simulink library "Pitch_Functions"  (Simulink 6.5)
undefined symbols (not defined in the file or in its folder): A, ABS, B, C, D, P_PitchProfilerAccLim, P_PitchProfilerMaxGain, P_PitchProfilerPostDelay, P_PitchProfilerPreDelay, P_PitchProfilerSpdLim, P_PitchProfilerTc, P_PitchProfilerTcRatio, P_PitchSpinningPos, PITCH_CYCLE_TIME, RND, SQR
libraries: StandardLib x187, WindLib x15, Pitch_Functions x6, simulink x4
(part 2 of 3)

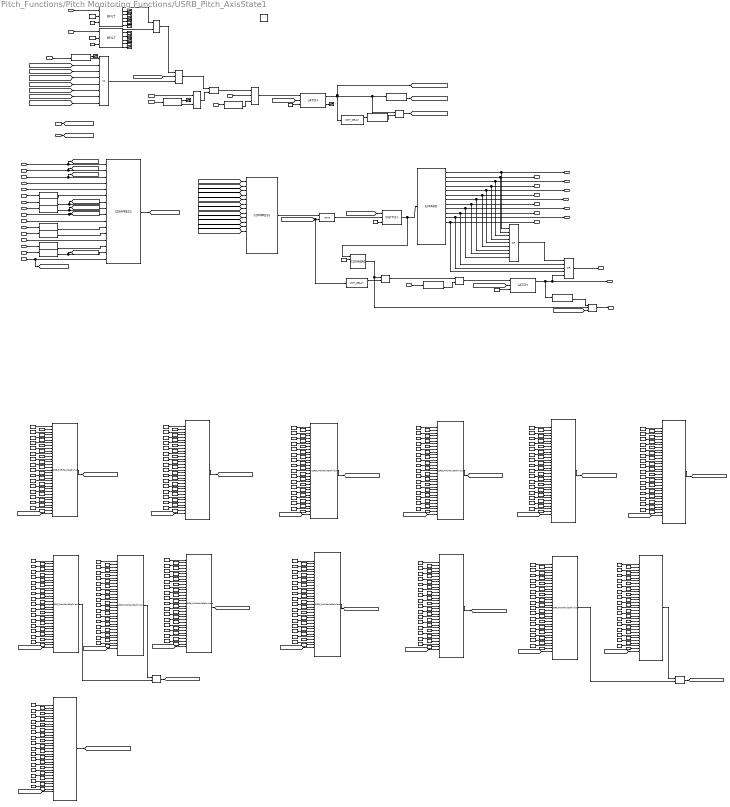
== system Pitch_Functions/Pitch Monitoring Functions/USRB_Pitch_AxisState1 ==
  note: Fault 11
  note: Fault 10
  note: Fault 9
  note: Fault 8
  note: Fault 7
  note: Fault 6
  note: Fault 5
  note: Fault 4
  note: Fault 3
  note: Fault 2
  note: Fault 1
  note: Fault 12
  B_In_SafetyLoopClosed : Inport  DataType=boolean
  DO_OpCtl_TbPitchRectifierOn : Inport  Port=2  DataType=boolean
  B_Pitch_ConverterReady : Inport  Port=3  DataType=boolean
  B_ResetLatch : Inport  Port=4  DataType=boolean
  B_EnableThyristorFault : Inport  Port=5  DataType=boolean
  B_Pitch_PitchThysitor : Inport  Port=6  DataType=boolean
  DI_In_PitchCtrlReady : Inport  Port=7  DataType=boolean
  DI_In_SpeedLoss : Inport  Port=8  DataType=boolean
  DI_In_MarkerLoss : Inport  Port=9  DataType=boolean
  DI_In_IncEncCorrection : Inport  Port=10  DataType=boolean
  DI_In_LS90AngleErr : Inport  Port=11  DataType=boolean
  DI_In_BatDCMCtr : Inport  Port=12  DataType=boolean
  DI_In_DCLinkOK : Inport  Port=13  DataType=boolean
  DI_In_BrakeOK : Inport  Port=14  DataType=boolean
  DI_In_FieldOK : Inport  Port=15  DataType=boolean
  DI_In_OverSpeed : Inport  Port=16  DataType=boolean
  DI_In_SpeedProfileFault : Inport  Port=17  DataType=boolean
  DI_In_SafetyRelayPLC : Inport  Port=18  DataType=boolean
  DI_In_CvrtDCMCtr : Inport  Port=19  DataType=boolean
  DI_In_LVRTAmpHourTrip : Inport  Port=20  DataType=boolean
  DI_In_PICCommOK : Inport  Port=21  DataType=boolean
  DI_In_PhaseOk : Inport  Port=22  DataType=boolean
  DI_In_CommunAEPAx_Ok : Inport  Port=23  DataType=boolean
  SM_Pitch_IOLinkAxisXFault : Inport  Port=24  DataType=boolean
  DI_In_ConverterFaulted : Inport  Port=25  DataType=boolean
  SM_Pitch_AxisxCtlUnitERR : Inport  Port=26  DataType=boolean
  1700ms : Constant  Value=1700  OutDataTypeMode=uint32  OutDataType=sfix(16)  ConRadixGroup=Use specified scaling  OutScaling=2^0  SampleTime=inf  FramePeriod=inf
  2h{1,19,30,32,34,36,40..43,45..46,48..58,60..61,63..71,74,76..78,81,83,88,91,94..95,97..98,100..106,108..109,112..118,120,126,132,134,137,140..141,143..144,146..152,154,168..169,171,174..175,177..178,180..183,185,195,198..199,202,205..209,214..222,224,226,229..235,237..238,240,248,253,256,259..264,266..273,275,280,282,290,292,294,297..301,305,307..312,326,337,342..346,348,364..365,368,372..376,384,386..387,390..393,398,405,409..410,412..416,418..424,426,431,438,440,443,446..450,486..492,494,505,508,511,514..515,517..518} (220 alike) : Constant  Value=1  OutDataTypeMode=boolean  OutDataType=sfix(16)  ConRadixGroup=Use specified scaling  OutScaling=2^0  SampleTime=inf  FramePeriod=inf
  2h{2..5,7..10,12..18,20..22,24..29,31,33,35,37..39,44,47,59,62,72..73,75,79,82,84..87,89..90,92..93,96,99,107,110..111,119,121..125,127..131,133,135..136,138..139,142,145,153,155..167,170,172..173,176,179,184,186..194,196..197,200..201,203..204,210..213,223,225,227..228,236,239,241..247,249..252,254..255,257..258,265,274,276..279,281,283..289,291,293,295..296,302..304,306,313..314,325,347,349,351..355,357..358,360..363,366..367,369..371,377..383,385,388..389,394..395,397,399..404,406..408,411,417,425,428..430,433..437,439,441..442,444..445,451..452,493,496..499,501..504,506..507,509..510,512..513,516,519} (230 alike) : Constant  Value=0  OutDataTypeMode=boolean  OutDataType=sfix(16)  ConRadixGroup=Use specified scaling  OutScaling=2^0  SampleTime=inf  FramePeriod=inf
  2h11 : Constant  Value=0  OutDataTypeMode=uint32  OutDataType=sfix(16)  ConRadixGroup=Use specified scaling  OutScaling=2^0  SampleTime=inf  FramePeriod=inf
  2h23 : Constant  Value=0  OutDataTypeMode=uint16  OutDataType=sfix(16)  ConRadixGroup=Use specified scaling  OutScaling=2^0  SampleTime=inf  FramePeriod=inf
  2h6 : Constant  Value=0  OutDataTypeMode=uint16  OutDataType=sfix(16)  ConRadixGroup=Use specified scaling  OutScaling=2^0  SampleTime=inf  FramePeriod=inf
  2h80 : Constant  Value=0  OutDataTypeMode=uint32  OutDataType=sfix(16)  ConRadixGroup=Use specified scaling  OutScaling=2^0  SampleTime=inf  FramePeriod=inf
  700ms : Constant  Value=700  OutDataTypeMode=uint32  OutDataType=sfix(16)  ConRadixGroup=Use specified scaling  OutScaling=2^0  SampleTime=inf  FramePeriod=inf
  AND{1..2,5,7,9} (5 alike) : StandardLib/Logical operations/AND  RepeatCnt=1  SampleTime=-1  ExecutionOrder=0
  AND10 : StandardLib/Logical operations/AND  RepeatCnt=2  SampleTime=-1  ExecutionOrder=0
  AND6 : StandardLib/Logical operations/AND  RepeatCnt=2  SampleTime=-1  ExecutionOrder=0
  AND8 : StandardLib/Logical operations/AND  RepeatCnt=2  SampleTime=-1  ExecutionOrder=0
  BFILT1 : StandardLib/Filters/BFILT  SampleTime=-1  ExecutionOrder=0
  BFILT3 : StandardLib/Filters/BFILT  SampleTime=-1  ExecutionOrder=0
  COMPARE : StandardLib/Math operations/COMPARE  Equation===  DataType=UINT16  SampleTime=-1  ExecutionOrder=0
  COMPRESS : StandardLib/Memory operations/COMPRESS  RepeatCnt=16  SampleTime=-1  ExecutionOrder=0
  COMPRESS4 : StandardLib/Memory operations/COMPRESS  RepeatCnt=16  SampleTime=-1  ExecutionOrder=0
  DocBlock1 : simulink/Model-Wide Utilities/DocBlock  SystemSampleTime=-1  DocumentType=Text
  EXPAND : StandardLib/Memory operations/EXPAND  SampleTime=-1  ExecutionOrder=0
  LATCH2 : StandardLib/Logical operations/LATCH  SampleTime=-1  ExecutionOrder=0
  LATCH3 : StandardLib/Logical operations/LATCH  SampleTime=-1  ExecutionOrder=0
  MOVE : StandardLib/Memory operations/MOVE  DataType=UINT16  SampleTime=-1  ExecutionOrder=0
  NOT{,1,3..11,13..15} (14 alike) : StandardLib/Logical operations/NOT  SampleTime=-1  ExecutionOrder=0
  OR : StandardLib/Logical operations/OR  RepeatCnt=1  SampleTime=-1  ExecutionOrder=0
  OR1 : StandardLib/Logical operations/OR  RepeatCnt=1  SampleTime=-1  ExecutionOrder=0
  OR2 : StandardLib/Logical operations/OR  RepeatCnt=1  SampleTime=-1  ExecutionOrder=0
  OR3 : StandardLib/Logical operations/OR  RepeatCnt=7  SampleTime=-1  ExecutionOrder=0
  OR4 : StandardLib/Logical operations/OR  RepeatCnt=8  SampleTime=-1  ExecutionOrder=0
  OR5 : StandardLib/Logical operations/OR  RepeatCnt=4  SampleTime=-1  ExecutionOrder=0
  SWITCH1 : StandardLib/Memory operations/SWITCH  DataType=UINT16  SampleTime=-1  ExecutionOrder=0
  Terminator{1..13} (13 alike) : Terminator
  UNIT_DELAY : StandardLib/Memory operations/UNIT_DELAY  DataType=BOOLEAN  SampleTime=-1  ExecutionOrder=0
  UNIT_DELAY1 : StandardLib/Memory operations/UNIT_DELAY  DataType=BOOLEAN  SampleTime=-1  ExecutionOrder=0
  USRB_PitchFaultDefinition_ConverterBrakeOK : WindLib/USRB_PitchFaultDefinition  SystemSampleTime=-1
  USRB_PitchFaultDefinition_ConverterDCLinkOK : WindLib/USRB_PitchFaultDefinition  SystemSampleTime=-1
  USRB_PitchFaultDefinition_ConverterFieldOK : WindLib/USRB_PitchFaultDefinition  SystemSampleTime=-1
  USRB_PitchFaultDefinition_ConverterFieldOK2 : WindLib/USRB_PitchFaultDefinition  SystemSampleTime=-1
  USRB_PitchFaultDefinition_ConverterIncEncCorrection : WindLib/USRB_PitchFaultDefinition  SystemSampleTime=-1
  USRB_PitchFaultDefinition_ConverterLS90AngleErr : WindLib/USRB_PitchFaultDefinition  SystemSampleTime=-1
  USRB_PitchFaultDefinition_ConverterMarkerLoss : WindLib/USRB_PitchFaultDefinition  SystemSampleTime=-1
  USRB_PitchFaultDefinition_ConverterOverSpeed : WindLib/USRB_PitchFaultDefinition  SystemSampleTime=-1
  USRB_PitchFaultDefinition_ConverterPICCommOK : WindLib/USRB_PitchFaultDefinition  SystemSampleTime=-1
  USRB_PitchFaultDefinition_ConverterPhaseOk : WindLib/USRB_PitchFaultDefinition  SystemSampleTime=-1
  USRB_PitchFaultDefinition_ConverterPhaseOk2 : WindLib/USRB_PitchFaultDefinition  SystemSampleTime=-1
  USRB_PitchFaultDefinition_ConverterSafetyRelayPLC : WindLib/USRB_PitchFaultDefinition  SystemSampleTime=-1
  USRB_PitchFaultDefinition_ConverterSpeedLoss : WindLib/USRB_PitchFaultDefinition  SystemSampleTime=-1
  USRB_PitchFaultDefinition_ConverterSpeedProfileFault : WindLib/USRB_PitchFaultDefinition  SystemSampleTime=-1
  SM_Pitch_ConverterSpeedLoss : Outport  DataType=boolean
  SM_Pitch_ConverterMarkerLoss : Outport  Port=2  DataType=boolean
  SM_Pitch_ConverterIncEncCorrection : Outport  Port=3  DataType=boolean
  SM_Pitch_ConverterLS90AngleErr : Outport  Port=4  DataType=boolean
  SM_Pitch_ConverterDCLinkOK : Outport  Port=5  DataType=boolean
  SM_Pitch_ConverterBrakeOK : Outport  Port=6  DataType=boolean
  SM_Pitch_ConverterFieldOK : Outport  Port=7  DataType=boolean
  SM_Pitch_ConverterOverSpeed : Outport  Port=8  DataType=boolean
  SM_Pitch_ConverterSafetyRelayPLC : Outport  Port=9  DataType=boolean
  SM_Pitch_ConverterPICCommOK : Outport  Port=10  DataType=boolean
  SM_Pitch_ConverterPhaseOk : Outport  Port=11  DataType=boolean
  SM_Pitch_ConverterSpeedProfileFault : Outport  Port=12  DataType=boolean
  B_PitchAxisMalfunc_L : Outport  Port=13  DataType=boolean
  SM_Pitch_ThyristorFault : Outport  Port=14  DataType=boolean
  B_AnyPitchThyristorFault : Outport  Port=15  DataType=boolean
  wires:
  AND6/1 -> OR1/1
  OR3/1 -> AND6/3
  NOT1/2 -> OR3/1
  B_Pitch_ConverterReady/1 -> NOT1/1
  [DI_In_PhaseOk] -> OR3/8
  [DI_In_OverSpeed] -> OR3/7
  [DI_In_FieldOK] -> OR3/6
  [DI_In_BrakeOK] -> OR3/5
  [DI_In_IncEncCorrection] -> OR3/4
  [DI_In_MarkerLoss] -> OR3/3
  [DI_In_SpeedLoss] -> OR3/2
  [CurrentFaultCode] -> USRB_PitchFaultDefinition_ConverterPhaseOk2/33
  [CurrentFaultCode] -> USRB_PitchFaultDefinition_ConverterPhaseOk/33
  [CurrentFaultCode] -> USRB_PitchFaultDefinition_ConverterPICCommOK/33
  [CurrentFaultCode] -> USRB_PitchFaultDefinition_ConverterSafetyRelayPLC/33
  [CurrentFaultCode] -> USRB_PitchFaultDefinition_ConverterOverSpeed/33
  [CurrentFaultCode] -> USRB_PitchFaultDefinition_ConverterFieldOK2/33
  [CurrentFaultCode] -> USRB_PitchFaultDefinition_ConverterBrakeOK/33
  [CurrentFaultCode] -> USRB_PitchFaultDefinition_ConverterDCLinkOK/33
  [CurrentFaultCode] -> USRB_PitchFaultDefinition_ConverterLS90AngleErr/33
  [CurrentFaultCode] -> USRB_PitchFaultDefinition_ConverterIncEncCorrection/33
  [CurrentFaultCode] -> USRB_PitchFaultDefinition_ConverterMarkerLoss/33
  [CurrentFaultCode] -> USRB_PitchFaultDefinition_ConverterSpeedLoss/33
  USRB_PitchFaultDefinition_ConverterFieldOK/1 -> OR2/2
  OR2/1 -> [B_Pitch_ConverterFieldOK]
  USRB_PitchFaultDefinition_ConverterFieldOK2/1 -> OR2/1
  2h76/1 -> USRB_PitchFaultDefinition_ConverterFieldOK2/32
  2h192/1 -> USRB_PitchFaultDefinition_ConverterFieldOK2/31
  2h34/1 -> USRB_PitchFaultDefinition_ConverterFieldOK2/30
  2h190/1 -> USRB_PitchFaultDefinition_ConverterFieldOK2/29
  2h209/1 -> USRB_PitchFaultDefinition_ConverterFieldOK2/28
  2h187/1 -> USRB_PitchFaultDefinition_ConverterFieldOK2/27
  2h210/1 -> USRB_PitchFaultDefinition_ConverterFieldOK2/26
  2h188/1 -> USRB_PitchFaultDefinition_ConverterFieldOK2/25
  2h208/1 -> USRB_PitchFaultDefinition_ConverterFieldOK2/24
  2h184/1 -> USRB_PitchFaultDefinition_ConverterFieldOK2/23
  2h206/1 -> USRB_PitchFaultDefinition_ConverterFieldOK2/22
  2h203/1 -> USRB_PitchFaultDefinition_ConverterFieldOK2/21
  2h207/1 -> USRB_PitchFaultDefinition_ConverterFieldOK2/20
  2h204/1 -> USRB_PitchFaultDefinition_ConverterFieldOK2/19
  2h205/1 -> USRB_PitchFaultDefinition_ConverterFieldOK2/18
  2h201/1 -> USRB_PitchFaultDefinition_ConverterFieldOK2/17
  2h185/1 -> USRB_PitchFaultDefinition_ConverterFieldOK2/16
  2h198/1 -> USRB_PitchFaultDefinition_ConverterFieldOK2/15
  2h202/1 -> USRB_PitchFaultDefinition_ConverterFieldOK2/14
  2h200/1 -> USRB_PitchFaultDefinition_ConverterFieldOK2/13
  2h183/1 -> USRB_PitchFaultDefinition_ConverterFieldOK2/12
  2h197/1 -> USRB_PitchFaultDefinition_ConverterFieldOK2/11
  2h181/1 -> USRB_PitchFaultDefinition_ConverterFieldOK2/10
  2h195/1 -> USRB_PitchFaultDefinition_ConverterFieldOK2/9
  2h182/1 -> USRB_PitchFaultDefinition_ConverterFieldOK2/8
  2h196/1 -> USRB_PitchFaultDefinition_ConverterFieldOK2/7
  2h180/1 -> USRB_PitchFaultDefinition_ConverterFieldOK2/6
  2h194/1 -> USRB_PitchFaultDefinition_ConverterFieldOK2/5
  2h77/1 -> USRB_PitchFaultDefinition_ConverterFieldOK2/2
  2h199/1 -> USRB_PitchFaultDefinition_ConverterFieldOK2/4
  2h189/1 -> USRB_PitchFaultDefinition_ConverterFieldOK2/3
  2h193/1 -> USRB_PitchFaultDefinition_ConverterFieldOK2/1
  NOT15/2 -> AND10/1
  AND10/1 -> B_PitchAxisMalfunc_L/1
  [DI_In_ConverterFaulted] -> AND10/3
  AND9/1 -> LATCH3/1
  LATCH3/1 -> NOT15/1, SM_Pitch_ThyristorFault/1, OR5/5
  AND2/1 -> AND9/1
  NOT14/2 -> AND9/2
  SM_Pitch_AxisxCtlUnitERR/1 -> NOT14/1
  [B_ConverterFault_Combined_NOT] -> LATCH3/2
  2h452/1 -> LATCH3/3
  SM_Pitch_IOLinkAxisXFault/1 -> NOT13/1
  NOT13/2 -> AND8/3
  USRB_PitchFaultDefinition_ConverterPhaseOk2/1 -> OR/1
  USRB_PitchFaultDefinition_ConverterPhaseOk/1 -> OR/2
  2h419/1 -> USRB_PitchFaultDefinition_ConverterPhaseOk2/32
  2h433/1 -> USRB_PitchFaultDefinition_ConverterPhaseOk2/31
  2h418/1 -> USRB_PitchFaultDefinition_ConverterPhaseOk2/30
  2h431/1 -> USRB_PitchFaultDefinition_ConverterPhaseOk2/29
  2h450/1 -> USRB_PitchFaultDefinition_ConverterPhaseOk2/28
  2h428/1 -> USRB_PitchFaultDefinition_ConverterPhaseOk2/27
  2h451/1 -> USRB_PitchFaultDefinition_ConverterPhaseOk2/26
  2h429/1 -> USRB_PitchFaultDefinition_ConverterPhaseOk2/25
  2h449/1 -> USRB_PitchFaultDefinition_ConverterPhaseOk2/24
  2h425/1 -> USRB_PitchFaultDefinition_ConverterPhaseOk2/23
  2h447/1 -> USRB_PitchFaultDefinition_ConverterPhaseOk2/22
  2h444/1 -> USRB_PitchFaultDefinition_ConverterPhaseOk2/21
  2h448/1 -> USRB_PitchFaultDefinition_ConverterPhaseOk2/20
  2h445/1 -> USRB_PitchFaultDefinition_ConverterPhaseOk2/19
  2h446/1 -> USRB_PitchFaultDefinition_ConverterPhaseOk2/18
  2h442/1 -> USRB_PitchFaultDefinition_ConverterPhaseOk2/17
  2h426/1 -> USRB_PitchFaultDefinition_ConverterPhaseOk2/16
  2h439/1 -> USRB_PitchFaultDefinition_ConverterPhaseOk2/15
  2h443/1 -> USRB_PitchFaultDefinition_ConverterPhaseOk2/14
  2h441/1 -> USRB_PitchFaultDefinition_ConverterPhaseOk2/13
  2h424/1 -> USRB_PitchFaultDefinition_ConverterPhaseOk2/12
  2h438/1 -> USRB_PitchFaultDefinition_ConverterPhaseOk2/11
  2h422/1 -> USRB_PitchFaultDefinition_ConverterPhaseOk2/10
  2h436/1 -> USRB_PitchFaultDefinition_ConverterPhaseOk2/9
  2h423/1 -> USRB_PitchFaultDefinition_ConverterPhaseOk2/8
  2h437/1 -> USRB_PitchFaultDefinition_ConverterPhaseOk2/7
  2h421/1 -> USRB_PitchFaultDefinition_ConverterPhaseOk2/6
  2h435/1 -> USRB_PitchFaultDefinition_ConverterPhaseOk2/5
  2h420/1 -> USRB_PitchFaultDefinition_ConverterPhaseOk2/2
  2h440/1 -> USRB_PitchFaultDefinition_ConverterPhaseOk2/4
  2h430/1 -> USRB_PitchFaultDefinition_ConverterPhaseOk2/3
  2h434/1 -> USRB_PitchFaultDefinition_ConverterPhaseOk2/1
  2h267/1 -> USRB_PitchFaultDefinition_ConverterPhaseOk/32
  2h283/1 -> USRB_PitchFaultDefinition_ConverterPhaseOk/31
  2h266/1 -> USRB_PitchFaultDefinition_ConverterPhaseOk/30
  2h280/1 -> USRB_PitchFaultDefinition_ConverterPhaseOk/29
  2h301/1 -> USRB_PitchFaultDefinition_ConverterPhaseOk/28
  2h277/1 -> USRB_PitchFaultDefinition_ConverterPhaseOk/27
  2h302/1 -> USRB_PitchFaultDefinition_ConverterPhaseOk/26
  2h278/1 -> USRB_PitchFaultDefinition_ConverterPhaseOk/25
  2h300/1 -> USRB_PitchFaultDefinition_ConverterPhaseOk/24
  2h274/1 -> USRB_PitchFaultDefinition_ConverterPhaseOk/23
  2h298/1 -> USRB_PitchFaultDefinition_ConverterPhaseOk/22
  2h295/1 -> USRB_PitchFaultDefinition_ConverterPhaseOk/21
  2h299/1 -> USRB_PitchFaultDefinition_ConverterPhaseOk/20
  2h296/1 -> USRB_PitchFaultDefinition_ConverterPhaseOk/19
  2h297/1 -> USRB_PitchFaultDefinition_ConverterPhaseOk/18
  2h293/1 -> USRB_PitchFaultDefinition_ConverterPhaseOk/17
  2h275/1 -> USRB_PitchFaultDefinition_ConverterPhaseOk/16
  2h289/1 -> USRB_PitchFaultDefinition_ConverterPhaseOk/15
  2h294/1 -> USRB_PitchFaultDefinition_ConverterPhaseOk/14
  2h291/1 -> USRB_PitchFaultDefinition_ConverterPhaseOk/13
  2h273/1 -> USRB_PitchFaultDefinition_ConverterPhaseOk/12
  2h288/1 -> USRB_PitchFaultDefinition_ConverterPhaseOk/11
  2h271/1 -> USRB_PitchFaultDefinition_ConverterPhaseOk/10
  2h286/1 -> USRB_PitchFaultDefinition_ConverterPhaseOk/9
  2h272/1 -> USRB_PitchFaultDefinition_ConverterPhaseOk/8
  2h287/1 -> USRB_PitchFaultDefinition_ConverterPhaseOk/7
  2h269/1 -> USRB_PitchFaultDefinition_ConverterPhaseOk/6
  2h285/1 -> USRB_PitchFaultDefinition_ConverterPhaseOk/5
  2h268/1 -> USRB_PitchFaultDefinition_ConverterPhaseOk/2
  2h290/1 -> USRB_PitchFaultDefinition_ConverterPhaseOk/4
  2h279/1 -> USRB_PitchFaultDefinition_ConverterPhaseOk/3
  2h284/1 -> USRB_PitchFaultDefinition_ConverterPhaseOk/1
  USRB_PitchFaultDefinition_ConverterPICCommOK/1 -> [B_Pitch_ConverterPICCommOK]
  2h230/1 -> USRB_PitchFaultDefinition_ConverterPICCommOK/32
  2h245/1 -> USRB_PitchFaultDefinition_ConverterPICCommOK/31
  2h229/1 -> USRB_PitchFaultDefinition_ConverterPICCommOK/30
  2h243/1 -> USRB_PitchFaultDefinition_ConverterPICCommOK/29
  2h264/1 -> USRB_PitchFaultDefinition_ConverterPICCommOK/28
  2h240/1 -> USRB_PitchFaultDefinition_ConverterPICCommOK/27
  2h265/1 -> USRB_PitchFaultDefinition_ConverterPICCommOK/26
  2h241/1 -> USRB_PitchFaultDefinition_ConverterPICCommOK/25
  2h263/1 -> USRB_PitchFaultDefinition_ConverterPICCommOK/24
  2h236/1 -> USRB_PitchFaultDefinition_ConverterPICCommOK/23
  2h261/1 -> USRB_PitchFaultDefinition_ConverterPICCommOK/22
  2h257/1 -> USRB_PitchFaultDefinition_ConverterPICCommOK/21
  2h262/1 -> USRB_PitchFaultDefinition_ConverterPICCommOK/20
  2h258/1 -> USRB_PitchFaultDefinition_ConverterPICCommOK/19
  2h260/1 -> USRB_PitchFaultDefinition_ConverterPICCommOK/18
  2h255/1 -> USRB_PitchFaultDefinition_ConverterPICCommOK/17
  2h238/1 -> USRB_PitchFaultDefinition_ConverterPICCommOK/16
  2h252/1 -> USRB_PitchFaultDefinition_ConverterPICCommOK/15
  2h256/1 -> USRB_PitchFaultDefinition_ConverterPICCommOK/14
  2h254/1 -> USRB_PitchFaultDefinition_ConverterPICCommOK/13
  2h235/1 -> USRB_PitchFaultDefinition_ConverterPICCommOK/12
  2h251/1 -> USRB_PitchFaultDefinition_ConverterPICCommOK/11
  2h233/1 -> USRB_PitchFaultDefinition_ConverterPICCommOK/10
  2h249/1 -> USRB_PitchFaultDefinition_ConverterPICCommOK/9
  2h234/1 -> USRB_PitchFaultDefinition_ConverterPICCommOK/8
  2h250/1 -> USRB_PitchFaultDefinition_ConverterPICCommOK/7
  2h232/1 -> USRB_PitchFaultDefinition_ConverterPICCommOK/6
  2h247/1 -> USRB_PitchFaultDefinition_ConverterPICCommOK/5
  2h231/1 -> USRB_PitchFaultDefinition_ConverterPICCommOK/2
  2h253/1 -> USRB_PitchFaultDefinition_ConverterPICCommOK/4
  2h242/1 -> USRB_PitchFaultDefinition_ConverterPICCommOK/3
  2h246/1 -> USRB_PitchFaultDefinition_ConverterPICCommOK/1
  USRB_PitchFaultDefinition_ConverterSafetyRelayPLC/1 -> [B_Pitch_ConverterSafetyRelayPLC]
  2h217/1 -> USRB_PitchFaultDefinition_ConverterSafetyRelayPLC/32
  2h397/1 -> USRB_PitchFaultDefinition_ConverterSafetyRelayPLC/31
  2h216/1 -> USRB_PitchFaultDefinition_ConverterSafetyRelayPLC/30
  2h395/1 -> USRB_PitchFaultDefinition_ConverterSafetyRelayPLC/29
  2h416/1 -> USRB_PitchFaultDefinition_ConverterSafetyRelayPLC/28
  2h227/1 -> USRB_PitchFaultDefinition_ConverterSafetyRelayPLC/27
  2h417/1 -> USRB_PitchFaultDefinition_ConverterSafetyRelayPLC/26
  2h228/1 -> USRB_PitchFaultDefinition_ConverterSafetyRelayPLC/25
  2h415/1 -> USRB_PitchFaultDefinition_ConverterSafetyRelayPLC/24
  2h223/1 -> USRB_PitchFaultDefinition_ConverterSafetyRelayPLC/23
  2h413/1 -> USRB_PitchFaultDefinition_ConverterSafetyRelayPLC/22
  2h410/1 -> USRB_PitchFaultDefinition_ConverterSafetyRelayPLC/21
  2h414/1 -> USRB_PitchFaultDefinition_ConverterSafetyRelayPLC/20
  2h411/1 -> USRB_PitchFaultDefinition_ConverterSafetyRelayPLC/19
  2h412/1 -> USRB_PitchFaultDefinition_ConverterSafetyRelayPLC/18
  2h408/1 -> USRB_PitchFaultDefinition_ConverterSafetyRelayPLC/17
  2h224/1 -> USRB_PitchFaultDefinition_ConverterSafetyRelayPLC/16
  2h404/1 -> USRB_PitchFaultDefinition_ConverterSafetyRelayPLC/15
  2h409/1 -> USRB_PitchFaultDefinition_ConverterSafetyRelayPLC/14
  2h406/1 -> USRB_PitchFaultDefinition_ConverterSafetyRelayPLC/13
  2h222/1 -> USRB_PitchFaultDefinition_ConverterSafetyRelayPLC/12
  2h403/1 -> USRB_PitchFaultDefinition_ConverterSafetyRelayPLC/11
  2h220/1 -> USRB_PitchFaultDefinition_ConverterSafetyRelayPLC/10
  2h401/1 -> USRB_PitchFaultDefinition_ConverterSafetyRelayPLC/9
  2h221/1 -> USRB_PitchFaultDefinition_ConverterSafetyRelayPLC/8
  2h402/1 -> USRB_PitchFaultDefinition_ConverterSafetyRelayPLC/7
  2h219/1 -> USRB_PitchFaultDefinition_ConverterSafetyRelayPLC/6
  2h400/1 -> USRB_PitchFaultDefinition_ConverterSafetyRelayPLC/5
  2h218/1 -> USRB_PitchFaultDefinition_ConverterSafetyRelayPLC/2
  2h405/1 -> USRB_PitchFaultDefinition_ConverterSafetyRelayPLC/4
  2h394/1 -> USRB_PitchFaultDefinition_ConverterSafetyRelayPLC/3
  2h399/1 -> USRB_PitchFaultDefinition_ConverterSafetyRelayPLC/1
  USRB_PitchFaultDefinition_ConverterOverSpeed/1 -> [B_Pitch_ConverterOverSpeed]
  2h215/1 -> USRB_PitchFaultDefinition_ConverterOverSpeed/32
  2h370/1 -> USRB_PitchFaultDefinition_ConverterOverSpeed/31
  2h214/1 -> USRB_PitchFaultDefinition_ConverterOverSpeed/30
  2h355/1 -> USRB_PitchFaultDefinition_ConverterOverSpeed/29
  2h398/1 -> USRB_PitchFaultDefinition_ConverterOverSpeed/28
  2h314/1 -> USRB_PitchFaultDefinition_ConverterOverSpeed/27
  2h407/1 -> USRB_PitchFaultDefinition_ConverterOverSpeed/26
  2h325/1 -> USRB_PitchFaultDefinition_ConverterOverSpeed/25
  2h393/1 -> USRB_PitchFaultDefinition_ConverterOverSpeed/24
  2h281/1 -> USRB_PitchFaultDefinition_ConverterOverSpeed/23
  2h391/1 -> USRB_PitchFaultDefinition_ConverterOverSpeed/22
  2h388/1 -> USRB_PitchFaultDefinition_ConverterOverSpeed/21
  2h392/1 -> USRB_PitchFaultDefinition_ConverterOverSpeed/20
  2h389/1 -> USRB_PitchFaultDefinition_ConverterOverSpeed/19
  2h390/1 -> USRB_PitchFaultDefinition_ConverterOverSpeed/18
  2h386/1 -> USRB_PitchFaultDefinition_ConverterOverSpeed/17
  2h292/1 -> USRB_PitchFaultDefinition_ConverterOverSpeed/16
  2h383/1 -> USRB_PitchFaultDefinition_ConverterOverSpeed/15
  2h387/1 -> USRB_PitchFaultDefinition_ConverterOverSpeed/14
  2h385/1 -> USRB_PitchFaultDefinition_ConverterOverSpeed/13
  2h270/1 -> USRB_PitchFaultDefinition_ConverterOverSpeed/12
  2h382/1 -> USRB_PitchFaultDefinition_ConverterOverSpeed/11
  2h248/1 -> USRB_PitchFaultDefinition_ConverterOverSpeed/10
  2h380/1 -> USRB_PitchFaultDefinition_ConverterOverSpeed/9
  2h259/1 -> USRB_PitchFaultDefinition_ConverterOverSpeed/8
  2h381/1 -> USRB_PitchFaultDefinition_ConverterOverSpeed/7
  2h237/1 -> USRB_PitchFaultDefinition_ConverterOverSpeed/6
  2h379/1 -> USRB_PitchFaultDefinition_ConverterOverSpeed/5
  2h226/1 -> USRB_PitchFaultDefinition_ConverterOverSpeed/2
  2h384/1 -> USRB_PitchFaultDefinition_ConverterOverSpeed/4
  2h349/1 -> USRB_PitchFaultDefinition_ConverterOverSpeed/3
  2h378/1 -> USRB_PitchFaultDefinition_ConverterOverSpeed/1
  [CurrentFaultCode] -> USRB_PitchFaultDefinition_ConverterFieldOK/33
  2h337/1 -> USRB_PitchFaultDefinition_ConverterFieldOK/32
  2h357/1 -> USRB_PitchFaultDefinition_ConverterFieldOK/31
  2h326/1 -> USRB_PitchFaultDefinition_ConverterFieldOK/30
  2h354/1 -> USRB_PitchFaultDefinition_ConverterFieldOK/29
  2h376/1 -> USRB_PitchFaultDefinition_ConverterFieldOK/28
  2h351/1 -> USRB_PitchFaultDefinition_ConverterFieldOK/27
  2h377/1 -> USRB_PitchFaultDefinition_ConverterFieldOK/26
  2h352/1 -> USRB_PitchFaultDefinition_ConverterFieldOK/25
  2h375/1 -> USRB_PitchFaultDefinition_ConverterFieldOK/24
  2h347/1 -> USRB_PitchFaultDefinition_ConverterFieldOK/23
  2h373/1 -> USRB_PitchFaultDefinition_ConverterFieldOK/22
  2h369/1 -> USRB_PitchFaultDefinition_ConverterFieldOK/21
  2h374/1 -> USRB_PitchFaultDefinition_ConverterFieldOK/20
  2h371/1 -> USRB_PitchFaultDefinition_ConverterFieldOK/19
  2h372/1 -> USRB_PitchFaultDefinition_ConverterFieldOK/18
  2h367/1 -> USRB_PitchFaultDefinition_ConverterFieldOK/17
  2h348/1 -> USRB_PitchFaultDefinition_ConverterFieldOK/16
  2h364/1 -> USRB_PitchFaultDefinition_ConverterFieldOK/15
  2h368/1 -> USRB_PitchFaultDefinition_ConverterFieldOK/14
  2h366/1 -> USRB_PitchFaultDefinition_ConverterFieldOK/13
  2h346/1 -> USRB_PitchFaultDefinition_ConverterFieldOK/12
  2h363/1 -> USRB_PitchFaultDefinition_ConverterFieldOK/11
  2h344/1 -> USRB_PitchFaultDefinition_ConverterFieldOK/10
  2h361/1 -> USRB_PitchFaultDefinition_ConverterFieldOK/9
  2h345/1 -> USRB_PitchFaultDefinition_ConverterFieldOK/8
  2h362/1 -> USRB_PitchFaultDefinition_ConverterFieldOK/7
  2h343/1 -> USRB_PitchFaultDefinition_ConverterFieldOK/6
  2h360/1 -> USRB_PitchFaultDefinition_ConverterFieldOK/5
  2h342/1 -> USRB_PitchFaultDefinition_ConverterFieldOK/2
  2h365/1 -> USRB_PitchFaultDefinition_ConverterFieldOK/4
  2h353/1 -> USRB_PitchFaultDefinition_ConverterFieldOK/3
  2h358/1 -> USRB_PitchFaultDefinition_ConverterFieldOK/1
  USRB_PitchFaultDefinition_ConverterBrakeOK/1 -> [B_Pitch_ConverterBrakeOK]
  2h147/1 -> USRB_PitchFaultDefinition_ConverterBrakeOK/32
  2h161/1 -> USRB_PitchFaultDefinition_ConverterBrakeOK/31
  2h146/1 -> USRB_PitchFaultDefinition_ConverterBrakeOK/30
  2h159/1 -> USRB_PitchFaultDefinition_ConverterBrakeOK/29
  2h178/1 -> USRB_PitchFaultDefinition_ConverterBrakeOK/28
  2h156/1 -> USRB_PitchFaultDefinition_ConverterBrakeOK/27
  2h179/1 -> USRB_PitchFaultDefinition_ConverterBrakeOK/26
  2h157/1 -> USRB_PitchFaultDefinition_ConverterBrakeOK/25
  2h177/1 -> USRB_PitchFaultDefinition_ConverterBrakeOK/24
  2h153/1 -> USRB_PitchFaultDefinition_ConverterBrakeOK/23
  2h175/1 -> USRB_PitchFaultDefinition_ConverterBrakeOK/22
  2h172/1 -> USRB_PitchFaultDefinition_ConverterBrakeOK/21
  2h176/1 -> USRB_PitchFaultDefinition_ConverterBrakeOK/20
  2h173/1 -> USRB_PitchFaultDefinition_ConverterBrakeOK/19
  2h174/1 -> USRB_PitchFaultDefinition_ConverterBrakeOK/18
  2h170/1 -> USRB_PitchFaultDefinition_ConverterBrakeOK/17
  2h154/1 -> USRB_PitchFaultDefinition_ConverterBrakeOK/16
  2h167/1 -> USRB_PitchFaultDefinition_ConverterBrakeOK/15
  2h171/1 -> USRB_PitchFaultDefinition_ConverterBrakeOK/14
  2h169/1 -> USRB_PitchFaultDefinition_ConverterBrakeOK/13
  2h152/1 -> USRB_PitchFaultDefinition_ConverterBrakeOK/12
  2h166/1 -> USRB_PitchFaultDefinition_ConverterBrakeOK/11
  2h150/1 -> USRB_PitchFaultDefinition_ConverterBrakeOK/10
  2h164/1 -> USRB_PitchFaultDefinition_ConverterBrakeOK/9
  2h151/1 -> USRB_PitchFaultDefinition_ConverterBrakeOK/8
  2h165/1 -> USRB_PitchFaultDefinition_ConverterBrakeOK/7
  2h149/1 -> USRB_PitchFaultDefinition_ConverterBrakeOK/6
  2h163/1 -> USRB_PitchFaultDefinition_ConverterBrakeOK/5
  2h148/1 -> USRB_PitchFaultDefinition_ConverterBrakeOK/2
  2h168/1 -> USRB_PitchFaultDefinition_ConverterBrakeOK/4
  2h158/1 -> USRB_PitchFaultDefinition_ConverterBrakeOK/3
  2h162/1 -> USRB_PitchFaultDefinition_ConverterBrakeOK/1
  USRB_PitchFaultDefinition_ConverterDCLinkOK/1 -> [B_Pitch_ConverterDCLinkOK]
  2h113/1 -> USRB_PitchFaultDefinition_ConverterDCLinkOK/32
  2h127/1 -> USRB_PitchFaultDefinition_ConverterDCLinkOK/31
  2h112/1 -> USRB_PitchFaultDefinition_ConverterDCLinkOK/30
  2h125/1 -> USRB_PitchFaultDefinition_ConverterDCLinkOK/29
  2h144/1 -> USRB_PitchFaultDefinition_ConverterDCLinkOK/28
  2h122/1 -> USRB_PitchFaultDefinition_ConverterDCLinkOK/27
  2h145/1 -> USRB_PitchFaultDefinition_ConverterDCLinkOK/26
  2h123/1 -> USRB_PitchFaultDefinition_ConverterDCLinkOK/25
  2h143/1 -> USRB_PitchFaultDefinition_ConverterDCLinkOK/24
  2h119/1 -> USRB_PitchFaultDefinition_ConverterDCLinkOK/23
  2h141/1 -> USRB_PitchFaultDefinition_ConverterDCLinkOK/22
  2h138/1 -> USRB_PitchFaultDefinition_ConverterDCLinkOK/21
  2h142/1 -> USRB_PitchFaultDefinition_ConverterDCLinkOK/20
  2h139/1 -> USRB_PitchFaultDefinition_ConverterDCLinkOK/19
  2h140/1 -> USRB_PitchFaultDefinition_ConverterDCLinkOK/18
  2h136/1 -> USRB_PitchFaultDefinition_ConverterDCLinkOK/17
  2h120/1 -> USRB_PitchFaultDefinition_ConverterDCLinkOK/16
  2h133/1 -> USRB_PitchFaultDefinition_ConverterDCLinkOK/15
  2h137/1 -> USRB_PitchFaultDefinition_ConverterDCLinkOK/14
  2h135/1 -> USRB_PitchFaultDefinition_ConverterDCLinkOK/13
  2h118/1 -> USRB_PitchFaultDefinition_ConverterDCLinkOK/12
  2h132/1 -> USRB_PitchFaultDefinition_ConverterDCLinkOK/11
  2h116/1 -> USRB_PitchFaultDefinition_ConverterDCLinkOK/10
  2h130/1 -> USRB_PitchFaultDefinition_ConverterDCLinkOK/9
  2h117/1 -> USRB_PitchFaultDefinition_ConverterDCLinkOK/8
  2h131/1 -> USRB_PitchFaultDefinition_ConverterDCLinkOK/7
  2h115/1 -> USRB_PitchFaultDefinition_ConverterDCLinkOK/6
  2h129/1 -> USRB_PitchFaultDefinition_ConverterDCLinkOK/5
  2h114/1 -> USRB_PitchFaultDefinition_ConverterDCLinkOK/2
  2h134/1 -> USRB_PitchFaultDefinition_ConverterDCLinkOK/4
  2h124/1 -> USRB_PitchFaultDefinition_ConverterDCLinkOK/3
  2h128/1 -> USRB_PitchFaultDefinition_ConverterDCLinkOK/1
  USRB_PitchFaultDefinition_ConverterLS90AngleErr/1 -> [B_Pitch_ConverterLS90AngleErr]
  2h487/1 -> USRB_PitchFaultDefinition_ConverterLS90AngleErr/32
  2h501/1 -> USRB_PitchFaultDefinition_ConverterLS90AngleErr/31
  2h486/1 -> USRB_PitchFaultDefinition_ConverterLS90AngleErr/30
  2h499/1 -> USRB_PitchFaultDefinition_ConverterLS90AngleErr/29
  2h518/1 -> USRB_PitchFaultDefinition_ConverterLS90AngleErr/28
  2h496/1 -> USRB_PitchFaultDefinition_ConverterLS90AngleErr/27
  2h519/1 -> USRB_PitchFaultDefinition_ConverterLS90AngleErr/26
  2h497/1 -> USRB_PitchFaultDefinition_ConverterLS90AngleErr/25
  2h517/1 -> USRB_PitchFaultDefinition_ConverterLS90AngleErr/24
  2h493/1 -> USRB_PitchFaultDefinition_ConverterLS90AngleErr/23
  2h515/1 -> USRB_PitchFaultDefinition_ConverterLS90AngleErr/22
  2h512/1 -> USRB_PitchFaultDefinition_ConverterLS90AngleErr/21
  2h516/1 -> USRB_PitchFaultDefinition_ConverterLS90AngleErr/20
  2h513/1 -> USRB_PitchFaultDefinition_ConverterLS90AngleErr/19
  2h514/1 -> USRB_PitchFaultDefinition_ConverterLS90AngleErr/18
  2h510/1 -> USRB_PitchFaultDefinition_ConverterLS90AngleErr/17
  2h494/1 -> USRB_PitchFaultDefinition_ConverterLS90AngleErr/16
  2h507/1 -> USRB_PitchFaultDefinition_ConverterLS90AngleErr/15
  2h511/1 -> USRB_PitchFaultDefinition_ConverterLS90AngleErr/14
  2h509/1 -> USRB_PitchFaultDefinition_ConverterLS90AngleErr/13
  2h492/1 -> USRB_PitchFaultDefinition_ConverterLS90AngleErr/12
  2h506/1 -> USRB_PitchFaultDefinition_ConverterLS90AngleErr/11
  2h490/1 -> USRB_PitchFaultDefinition_ConverterLS90AngleErr/10
  2h504/1 -> USRB_PitchFaultDefinition_ConverterLS90AngleErr/9
  2h491/1 -> USRB_PitchFaultDefinition_ConverterLS90AngleErr/8
  2h505/1 -> USRB_PitchFaultDefinition_ConverterLS90AngleErr/7
  2h489/1 -> USRB_PitchFaultDefinition_ConverterLS90AngleErr/6
  2h503/1 -> USRB_PitchFaultDefinition_ConverterLS90AngleErr/5
  2h488/1 -> USRB_PitchFaultDefinition_ConverterLS90AngleErr/2
  2h508/1 -> USRB_PitchFaultDefinition_ConverterLS90AngleErr/4
  2h498/1 -> USRB_PitchFaultDefinition_ConverterLS90AngleErr/3
  2h502/1 -> USRB_PitchFaultDefinition_ConverterLS90AngleErr/1
  USRB_PitchFaultDefinition_ConverterIncEncCorrection/1 -> [B_Pitch_ConverterIncEncCorrection]
  2h101/1 -> USRB_PitchFaultDefinition_ConverterIncEncCorrection/32
  2h75/1 -> USRB_PitchFaultDefinition_ConverterIncEncCorrection/31
  2h100/1 -> USRB_PitchFaultDefinition_ConverterIncEncCorrection/30
  2h73/1 -> USRB_PitchFaultDefinition_ConverterIncEncCorrection/29
  2h98/1 -> USRB_PitchFaultDefinition_ConverterIncEncCorrection/28
  2h110/1 -> USRB_PitchFaultDefinition_ConverterIncEncCorrection/27
  2h99/1 -> USRB_PitchFaultDefinition_ConverterIncEncCorrection/26
  2h111/1 -> USRB_PitchFaultDefinition_ConverterIncEncCorrection/25
  2h97/1 -> USRB_PitchFaultDefinition_ConverterIncEncCorrection/24
  2h107/1 -> USRB_PitchFaultDefinition_ConverterIncEncCorrection/23
  2h95/1 -> USRB_PitchFaultDefinition_ConverterIncEncCorrection/22
  2h92/1 -> USRB_PitchFaultDefinition_ConverterIncEncCorrection/21
  2h96/1 -> USRB_PitchFaultDefinition_ConverterIncEncCorrection/20
  2h93/1 -> USRB_PitchFaultDefinition_ConverterIncEncCorrection/19
  2h94/1 -> USRB_PitchFaultDefinition_ConverterIncEncCorrection/18
  2h90/1 -> USRB_PitchFaultDefinition_ConverterIncEncCorrection/17
  2h108/1 -> USRB_PitchFaultDefinition_ConverterIncEncCorrection/16
  2h87/1 -> USRB_PitchFaultDefinition_ConverterIncEncCorrection/15
  2h91/1 -> USRB_PitchFaultDefinition_ConverterIncEncCorrection/14
  2h89/1 -> USRB_PitchFaultDefinition_ConverterIncEncCorrection/13
  2h106/1 -> USRB_PitchFaultDefinition_ConverterIncEncCorrection/12
  2h86/1 -> USRB_PitchFaultDefinition_ConverterIncEncCorrection/11
  2h104/1 -> USRB_PitchFaultDefinition_ConverterIncEncCorrection/10
  2h84/1 -> USRB_PitchFaultDefinition_ConverterIncEncCorrection/9
  2h105/1 -> USRB_PitchFaultDefinition_ConverterIncEncCorrection/8
  2h85/1 -> USRB_PitchFaultDefinition_ConverterIncEncCorrection/7
  2h103/1 -> USRB_PitchFaultDefinition_ConverterIncEncCorrection/6
  2h83/1 -> USRB_PitchFaultDefinition_ConverterIncEncCorrection/5
  2h102/1 -> USRB_PitchFaultDefinition_ConverterIncEncCorrection/2
  2h88/1 -> USRB_PitchFaultDefinition_ConverterIncEncCorrection/4
  2h72/1 -> USRB_PitchFaultDefinition_ConverterIncEncCorrection/3
  2h82/1 -> USRB_PitchFaultDefinition_ConverterIncEncCorrection/1
  USRB_PitchFaultDefinition_ConverterMarkerLoss/1 -> [B_Pitch_ConverterMarkerLoss]
  2h64/1 -> USRB_PitchFaultDefinition_ConverterMarkerLoss/32
  2h12/1 -> USRB_PitchFaultDefinition_ConverterMarkerLoss/31
  2h63/1 -> USRB_PitchFaultDefinition_ConverterMarkerLoss/30
  2h10/1 -> USRB_PitchFaultDefinition_ConverterMarkerLoss/29
  2h61/1 -> USRB_PitchFaultDefinition_ConverterMarkerLoss/28
  2h8/1 -> USRB_PitchFaultDefinition_ConverterMarkerLoss/27
  2h62/1 -> USRB_PitchFaultDefinition_ConverterMarkerLoss/26
  2h9/1 -> USRB_PitchFaultDefinition_ConverterMarkerLoss/25
  2h60/1 -> USRB_PitchFaultDefinition_ConverterMarkerLoss/24
  2h7/1 -> USRB_PitchFaultDefinition_ConverterMarkerLoss/23
  2h58/1 -> USRB_PitchFaultDefinition_ConverterMarkerLoss/22
  2h4/1 -> USRB_PitchFaultDefinition_ConverterMarkerLoss/21
  2h59/1 -> USRB_PitchFaultDefinition_ConverterMarkerLoss/20
  2h5/1 -> USRB_PitchFaultDefinition_ConverterMarkerLoss/19
  2h57/1 -> USRB_PitchFaultDefinition_ConverterMarkerLoss/18
  2h3/1 -> USRB_PitchFaultDefinition_ConverterMarkerLoss/17
  2h70/1 -> USRB_PitchFaultDefinition_ConverterMarkerLoss/16
  2h18/1 -> USRB_PitchFaultDefinition_ConverterMarkerLoss/15
  2h36/1 -> USRB_PitchFaultDefinition_ConverterMarkerLoss/14
  2h2/1 -> USRB_PitchFaultDefinition_ConverterMarkerLoss/13
  2h69/1 -> USRB_PitchFaultDefinition_ConverterMarkerLoss/12
  2h17/1 -> USRB_PitchFaultDefinition_ConverterMarkerLoss/11
  2h67/1 -> USRB_PitchFaultDefinition_ConverterMarkerLoss/10
  2h15/1 -> USRB_PitchFaultDefinition_ConverterMarkerLoss/9
  2h68/1 -> USRB_PitchFaultDefinition_ConverterMarkerLoss/8
  2h16/1 -> USRB_PitchFaultDefinition_ConverterMarkerLoss/7
  2h66/1 -> USRB_PitchFaultDefinition_ConverterMarkerLoss/6
  2h14/1 -> USRB_PitchFaultDefinition_ConverterMarkerLoss/5
  2h65/1 -> USRB_PitchFaultDefinition_ConverterMarkerLoss/2
  2h19/1 -> USRB_PitchFaultDefinition_ConverterMarkerLoss/4
  2h1/1 -> USRB_PitchFaultDefinition_ConverterMarkerLoss/3
  2h13/1 -> USRB_PitchFaultDefinition_ConverterMarkerLoss/1
  USRB_PitchFaultDefinition_ConverterSpeedLoss/1 -> [B_Pitch_ConverterSpeedLoss]
  2h49/1 -> USRB_PitchFaultDefinition_ConverterSpeedLoss/32
  2h31/1 -> USRB_PitchFaultDefinition_ConverterSpeedLoss/31
  2h48/1 -> USRB_PitchFaultDefinition_ConverterSpeedLoss/30
  2h29/1 -> USRB_PitchFaultDefinition_ConverterSpeedLoss/29
  2h46/1 -> USRB_PitchFaultDefinition_ConverterSpeedLoss/28
  2h27/1 -> USRB_PitchFaultDefinition_ConverterSpeedLoss/27
  2h47/1 -> USRB_PitchFaultDefinition_ConverterSpeedLoss/26
  2h28/1 -> USRB_PitchFaultDefinition_ConverterSpeedLoss/25
  2h45/1 -> USRB_PitchFaultDefinition_ConverterSpeedLoss/24
  2h26/1 -> USRB_PitchFaultDefinition_ConverterSpeedLoss/23
  2h43/1 -> USRB_PitchFaultDefinition_ConverterSpeedLoss/22
  2h24/1 -> USRB_PitchFaultDefinition_ConverterSpeedLoss/21
  2h44/1 -> USRB_PitchFaultDefinition_ConverterSpeedLoss/20
  2h25/1 -> USRB_PitchFaultDefinition_ConverterSpeedLoss/19
  2h42/1 -> USRB_PitchFaultDefinition_ConverterSpeedLoss/18
  2h22/1 -> USRB_PitchFaultDefinition_ConverterSpeedLoss/17
  2h55/1 -> USRB_PitchFaultDefinition_ConverterSpeedLoss/16
  2h39/1 -> USRB_PitchFaultDefinition_ConverterSpeedLoss/15
  2h41/1 -> USRB_PitchFaultDefinition_ConverterSpeedLoss/14
  2h21/1 -> USRB_PitchFaultDefinition_ConverterSpeedLoss/13
  2h54/1 -> USRB_PitchFaultDefinition_ConverterSpeedLoss/12
  2h38/1 -> USRB_PitchFaultDefinition_ConverterSpeedLoss/11
  2h52/1 -> USRB_PitchFaultDefinition_ConverterSpeedLoss/10
  2h35/1 -> USRB_PitchFaultDefinition_ConverterSpeedLoss/9
  2h53/1 -> USRB_PitchFaultDefinition_ConverterSpeedLoss/8
  2h37/1 -> USRB_PitchFaultDefinition_ConverterSpeedLoss/7
  2h51/1 -> USRB_PitchFaultDefinition_ConverterSpeedLoss/6
  2h33/1 -> USRB_PitchFaultDefinition_ConverterSpeedLoss/5
  DI_In_ConverterFaulted/1 -> COMPRESS/16, [DI_In_ConverterFaulted]
  DI_In_CommunAEPAx_Ok/1 -> AND8/2
  AND8/1 -> LATCH2/1
  OR1/1 -> AND8/1
  COMPRESS/1 -> [CurrentFaultCode]
  2h50/1 -> USRB_PitchFaultDefinition_ConverterSpeedLoss/2
  2h40/1 -> USRB_PitchFaultDefinition_ConverterSpeedLoss/4
  NOT11/2 -> [DI_In_PhaseOk], COMPRESS/15
  DI_In_PhaseOk/1 -> NOT11/1
  NOT10/2 -> COMPRESS/14
  DI_In_PICCommOK/1 -> NOT10/1
  NOT9/2 -> COMPRESS/12
  DI_In_CvrtDCMCtr/1 -> NOT9/1
  NOT8/2 -> COMPRESS/11
  DI_In_SafetyRelayPLC/1 -> NOT8/1
  NOT7/2 -> [DI_In_FieldOK], COMPRESS/8
  DI_In_FieldOK/1 -> NOT7/1
  NOT6/2 -> [DI_In_BrakeOK], COMPRESS/7
  DI_In_BrakeOK/1 -> NOT6/1
  NOT4/2 -> COMPRESS/6
  DI_In_DCLinkOK/1 -> NOT4/1
  OR/1 -> [B_Pitch_ConverterPhaseOk]
  [B_Pitch_ConverterPhaseOk] -> COMPRESS4/11
  [B_Pitch_ConverterPICCommOK] -> COMPRESS4/10
  [B_Pitch_ConverterSafetyRelayPLC] -> COMPRESS4/9
  [B_Pitch_ConverterOverSpeed] -> COMPRESS4/8
  [B_Pitch_ConverterFieldOK] -> COMPRESS4/7
  [B_Pitch_ConverterBrakeOK] -> COMPRESS4/6
  [B_Pitch_ConverterDCLinkOK] -> COMPRESS4/5
  [B_Pitch_ConverterLS90AngleErr] -> COMPRESS4/4
  [B_Pitch_ConverterIncEncCorrection] -> COMPRESS4/3
  [B_Pitch_ConverterMarkerLoss] -> COMPRESS4/2
  EXPAND/11 -> SM_Pitch_ConverterPhaseOk/1, OR5/3
  EXPAND/10 -> SM_Pitch_ConverterPICCommOK/1, OR5/2
  EXPAND/9 -> SM_Pitch_ConverterSafetyRelayPLC/1, OR4/9
  EXPAND/8 -> SM_Pitch_ConverterOverSpeed/1, OR4/8
  EXPAND/7 -> SM_Pitch_ConverterFieldOK/1, OR4/7
  EXPAND/6 -> SM_Pitch_ConverterBrakeOK/1, OR4/6
  EXPAND/5 -> SM_Pitch_ConverterDCLinkOK/1, OR4/5
  B_EnableThyristorFault/1 -> [B_EnableThyristorFault]
  B_ResetLatch/1 -> [B_ResetLatch]
  NOT3/2 -> [B_ConverterFault_Combined_NOT]
  AND1/1 -> [ConverterFault_CombinedPosEdge]
  UNIT_DELAY/1 -> NOT/1
  NOT/2 -> AND1/2
  700ms/1 -> BFILT3/2
  2h80/1 -> BFILT3/3
  2h79/1 -> LATCH2/3
  LATCH2/1 -> AND1/1, NOT3/1, [ConverterFault_Combined], UNIT_DELAY/1
  B_Pitch_PitchThysitor/1 -> AND7/1
  DI_In_PitchCtrlReady/1 -> NOT5/1
  NOT5/2 -> AND7/2
  [B_ResetLatch] -> LATCH2/2
  NOT1/1 -> Terminator5/1
  [B_EnableThyristorFault] -> AND6/2
  BFILT3/2 -> Terminator6/1
  BFILT3/3 -> Terminator7/1
  BFILT3/4 -> Terminator8/1
  BFILT3/5 -> Terminator9/1
  BFILT3/6 -> Terminator10/1
  AND7/1 -> OR1/2
  NOT5/1 -> Terminator4/1
  LATCH2/2 -> Terminator11/1
  2h20/1 -> USRB_PitchFaultDefinition_ConverterSpeedLoss/3
  2h32/1 -> USRB_PitchFaultDefinition_ConverterSpeedLoss/1
  UNIT_DELAY1/1 -> AND2/2
  COMPARE/1 -> AND10/2, AND2/1
  2h6/1 -> COMPARE/2
  [B_Pitch_ConverterSpeedLoss] -> COMPRESS4/1
  MOVE/1 -> SWITCH1/2
  [ConverterFault_CombinedPosEdge] -> UNIT_DELAY1/1, MOVE/2
  COMPRESS4/1 -> MOVE/1
  EXPAND/4 -> SM_Pitch_ConverterLS90AngleErr/1, OR4/4
  EXPAND/3 -> SM_Pitch_ConverterIncEncCorrection/1, OR4/3
  EXPAND/2 -> SM_Pitch_ConverterMarkerLoss/1, OR4/2
  2h23/1 -> SWITCH1/3
  [ConverterFault_Combined] -> SWITCH1/1
  SWITCH1/1 -> COMPARE/1, EXPAND/1
  EXPAND/1 -> SM_Pitch_ConverterSpeedLoss/1, OR4/1
  DI_In_LVRTAmpHourTrip/1 -> COMPRESS/13
  DI_In_SpeedProfileFault/1 -> COMPRESS/10
  DI_In_OverSpeed/1 -> [DI_In_OverSpeed], COMPRESS/9
  DI_In_BatDCMCtr/1 -> COMPRESS/5
  DI_In_LS90AngleErr/1 -> COMPRESS/4
  DI_In_IncEncCorrection/1 -> [DI_In_IncEncCorrection], COMPRESS/3
  DI_In_MarkerLoss/1 -> [DI_In_MarkerLoss], COMPRESS/2
  DI_In_SpeedLoss/1 -> [DI_In_SpeedLoss], COMPRESS/1
  OR4/1 -> OR5/1
  OR5/1 -> B_AnyPitchThyristorFault/1
  B_In_SafetyLoopClosed/1 -> BFILT1/1
  1700ms/1 -> BFILT1/2
  2h11/1 -> BFILT1/3
  BFILT1/1 -> AND5/1
  BFILT1/2 -> Terminator2/1
  BFILT1/3 -> Terminator3/1
  BFILT1/4 -> Terminator12/1
  BFILT1/5 -> Terminator13/1
  BFILT1/6 -> Terminator1/1
  BFILT3/1 -> AND5/2
  DO_OpCtl_TbPitchRectifierOn/1 -> BFILT3/1
  AND5/1 -> AND6/1
  [CurrentFaultCode] -> USRB_PitchFaultDefinition_ConverterSpeedProfileFault/33
  USRB_PitchFaultDefinition_ConverterSpeedProfileFault/1 -> [B_Pitch_ConverterSpeedProfileFault]
  2h56/1 -> USRB_PitchFaultDefinition_ConverterSpeedProfileFault/32
  2h211/1 -> USRB_PitchFaultDefinition_ConverterSpeedProfileFault/31
  2h30/1 -> USRB_PitchFaultDefinition_ConverterSpeedProfileFault/30
  2h191/1 -> USRB_PitchFaultDefinition_ConverterSpeedProfileFault/29
  2h312/1 -> USRB_PitchFaultDefinition_ConverterSpeedProfileFault/28
  2h155/1 -> USRB_PitchFaultDefinition_ConverterSpeedProfileFault/27
  2h313/1 -> USRB_PitchFaultDefinition_ConverterSpeedProfileFault/26
  2h160/1 -> USRB_PitchFaultDefinition_ConverterSpeedProfileFault/25
  2h311/1 -> USRB_PitchFaultDefinition_ConverterSpeedProfileFault/24
  2h121/1 -> USRB_PitchFaultDefinition_ConverterSpeedProfileFault/23
  2h309/1 -> USRB_PitchFaultDefinition_ConverterSpeedProfileFault/22
  2h306/1 -> USRB_PitchFaultDefinition_ConverterSpeedProfileFault/21
  2h310/1 -> USRB_PitchFaultDefinition_ConverterSpeedProfileFault/20
  2h307/1 -> USRB_PitchFaultDefinition_ConverterSpeedProfileFault/19
  2h308/1 -> USRB_PitchFaultDefinition_ConverterSpeedProfileFault/18
  2h304/1 -> USRB_PitchFaultDefinition_ConverterSpeedProfileFault/17
  2h126/1 -> USRB_PitchFaultDefinition_ConverterSpeedProfileFault/16
  2h276/1 -> USRB_PitchFaultDefinition_ConverterSpeedProfileFault/15
  2h305/1 -> USRB_PitchFaultDefinition_ConverterSpeedProfileFault/14
  2h303/1 -> USRB_PitchFaultDefinition_ConverterSpeedProfileFault/13
  2h109/1 -> USRB_PitchFaultDefinition_ConverterSpeedProfileFault/12
  2h244/1 -> USRB_PitchFaultDefinition_ConverterSpeedProfileFault/11
  2h78/1 -> USRB_PitchFaultDefinition_ConverterSpeedProfileFault/10
  2h225/1 -> USRB_PitchFaultDefinition_ConverterSpeedProfileFault/9
  2h81/1 -> USRB_PitchFaultDefinition_ConverterSpeedProfileFault/8
  2h239/1 -> USRB_PitchFaultDefinition_ConverterSpeedProfileFault/7
  2h74/1 -> USRB_PitchFaultDefinition_ConverterSpeedProfileFault/6
  2h213/1 -> USRB_PitchFaultDefinition_ConverterSpeedProfileFault/5
  2h71/1 -> USRB_PitchFaultDefinition_ConverterSpeedProfileFault/2
  2h282/1 -> USRB_PitchFaultDefinition_ConverterSpeedProfileFault/4
  2h186/1 -> USRB_PitchFaultDefinition_ConverterSpeedProfileFault/3
  2h212/1 -> USRB_PitchFaultDefinition_ConverterSpeedProfileFault/1
  [B_Pitch_ConverterSpeedProfileFault] -> COMPRESS4/12
  EXPAND/12 -> SM_Pitch_ConverterSpeedProfileFault/1, OR5/4

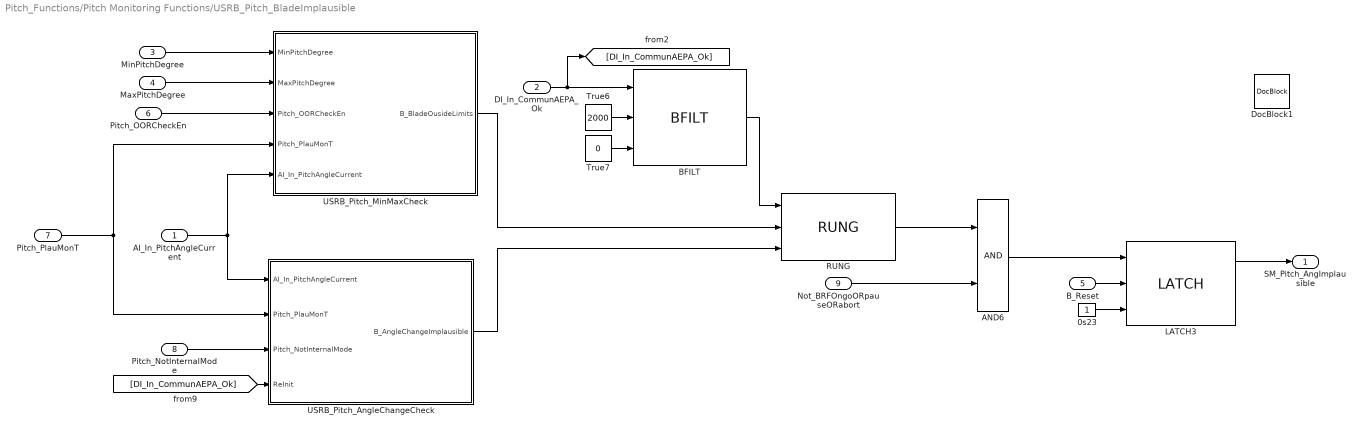
== system Pitch_Functions/Pitch Monitoring Functions/USRB_Pitch_BladeImplausible ==
  AI_In_PitchAngleCurrent : Inport  DataType=single
  DI_In_CommunAEPA_Ok : Inport  Port=2  DataType=boolean
      settings: BusObject=Outputs
  MinPitchDegree : Inport  Port=3  DataType=single
  MaxPitchDegree : Inport  Port=4  DataType=single
  B_Reset : Inport  Port=5  DataType=boolean
  Pitch_OORCheckEn : Inport  Port=6  DataType=boolean
  Pitch_PlauMonT : Inport  Port=7  DataType=uint32
  Pitch_NotInternalMode : Inport  Port=8  DataType=boolean
  Not_BRFOngoORpauseORabort : Inport  Port=9  DataType=boolean
  0s23 : Constant  Value=1  OutDataTypeMode=boolean  OutDataType=sfix(16)  ConRadixGroup=Use specified scaling  OutScaling=2^0  SampleTime=inf  FramePeriod=inf
  AND6 : StandardLib/Logical operations/AND  RepeatCnt=1  SampleTime=-1  ExecutionOrder=0
  BFILT : StandardLib/Filters/BFILT  SampleTime=-1  ExecutionOrder=0
  DocBlock1 : simulink/Model-Wide Utilities/DocBlock  SystemSampleTime=-1  DocumentType=Text
  LATCH3 : StandardLib/Logical operations/LATCH  SampleTime=-1  ExecutionOrder=0
  RUNG : StandardLib/Logical operations/RUNG  Equation=(A*(B+C))  RepeatCount=3  SampleTime=-1  ExecutionOrder=0
  True6 : Constant  Value=2000  OutDataTypeMode=uint32  OutDataType=sfix(16)  ConRadixGroup=Use specified scaling  OutScaling=2^0  SampleTime=-1  FramePeriod=inf
  True7 : Constant  Value=0  OutDataTypeMode=uint32  OutDataType=sfix(16)  ConRadixGroup=Use specified scaling  OutScaling=2^0  SampleTime=-1  FramePeriod=inf
  USRB_Pitch_AngleChangeCheck : Subsystem  TreatAsAtomicUnit=on
  USRB_Pitch_MinMaxCheck : Subsystem  TreatAsAtomicUnit=on
  SM_Pitch_AngImplausible : Outport  DataType=boolean
  wires:
  0s23/1 -> LATCH3/3
  USRB_Pitch_MinMaxCheck/1(B_BladeOusideLimits) -> RUNG/2
  USRB_Pitch_AngleChangeCheck/1(B_AngleChangeImplausible) -> RUNG/3
  B_Reset/1 -> LATCH3/2
  LATCH3/1 -> SM_Pitch_AngImplausible/1
  AI_In_PitchAngleCurrent/1 -> USRB_Pitch_MinMaxCheck/5(AI_In_PitchAngleCurrent), USRB_Pitch_AngleChangeCheck/1(AI_In_PitchAngleCurrent)
  MinPitchDegree/1 -> USRB_Pitch_MinMaxCheck/1(MinPitchDegree)
  MaxPitchDegree/1 -> USRB_Pitch_MinMaxCheck/2(MaxPitchDegree)
  Pitch_NotInternalMode/1 -> USRB_Pitch_AngleChangeCheck/3(Pitch_NotInternalMode)
  Pitch_OORCheckEn/1 -> USRB_Pitch_MinMaxCheck/3(Pitch_OORCheckEn)
  Pitch_PlauMonT/1 -> USRB_Pitch_MinMaxCheck/4(Pitch_PlauMonT), USRB_Pitch_AngleChangeCheck/2(Pitch_PlauMonT)
  DI_In_CommunAEPA_Ok/1 -> BFILT/1, [DI_In_CommunAEPA_Ok]
  True6/1 -> BFILT/2
  True7/1 -> BFILT/3
  BFILT/1 -> RUNG/1
  Not_BRFOngoORpauseORabort/1 -> AND6/2
  RUNG/1 -> AND6/1
  AND6/1 -> LATCH3/1
  [DI_In_CommunAEPA_Ok] -> USRB_Pitch_AngleChangeCheck/4(ReInit)

== system Pitch_Functions/Pitch Monitoring Functions/USRB_Pitch_BladePitching ==
  note: ***********************************************************************************************************************************************
      | ***********         Change history. Please include your changes below and in the in the modified Task / USRB         ***********
      | ***********************************************************************************************************************************************
      |
      | 2013-01-31, JGC: Corrected logic of Pitching time to long. During EBST of one blade do not monitor the other to axis
  B_MaxBattPitchingTimePass_LL : Inport  DataType=boolean
  PitchAngleCurrent : Inport  Port=2  DataType=single
  B_Pitch_90DegLimitSwitch : Inport  Port=3  DataType=boolean
  AND1 : StandardLib/Logical operations/AND  RepeatCnt=2  SampleTime=-1  ExecutionOrder=0
  COMPARE : StandardLib/Math operations/COMPARE  Equation=<  DataType=SINGLE  SampleTime=-1  ExecutionOrder=0
  Constant : Constant  Value=1  OutDataTypeMode=single  OutDataType=sfix(16)  ConRadixGroup=Use specified scaling  OutScaling=2^0  SampleTime=-1  FramePeriod=inf
  DocBlock : simulink/Model-Wide Utilities/DocBlock  SystemSampleTime=-1  DocumentType=Text
  SUB : StandardLib/Math operations/SUB  DataType=SINGLE  SampleTime=-1  ExecutionOrder=0
  from17 : Constant  Value=P_PitchSpinningPos  OutDataTypeMode=single  OutDataType=sfix(16)  ConRadixGroup=Use specified scaling  OutScaling=2^0  SampleTime=inf  FramePeriod=inf
  B_BladePitchingLong_LL : Outport  DataType=boolean
  wires:
  B_MaxBattPitchingTimePass_LL/1 -> AND1/3
  B_Pitch_90DegLimitSwitch/1 -> AND1/2
  AND1/1 -> B_BladePitchingLong_LL/1
  PitchAngleCurrent/1 -> SUB/1
  Constant/1 -> SUB/2
  COMPARE/1 -> AND1/1
  from17/1 -> COMPARE/2
  SUB/1 -> COMPARE/1
